simulink subsystem "BranchDecisionLogic"  (R2024b)
settings: Solver=VariableStepAuto  StartTime=0.0  StopTime=10.0  RelTol=1e-3
libraries: hdlsllib x1
settings Model: Creator=stefano  LastModifiedBy=stefano

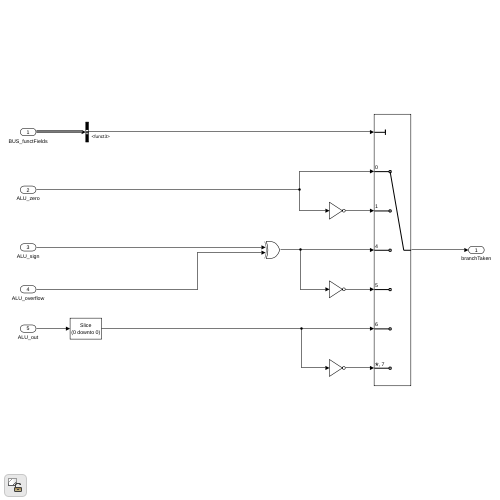
[thumbnail: Simulink's stored preview of the top-level diagram]
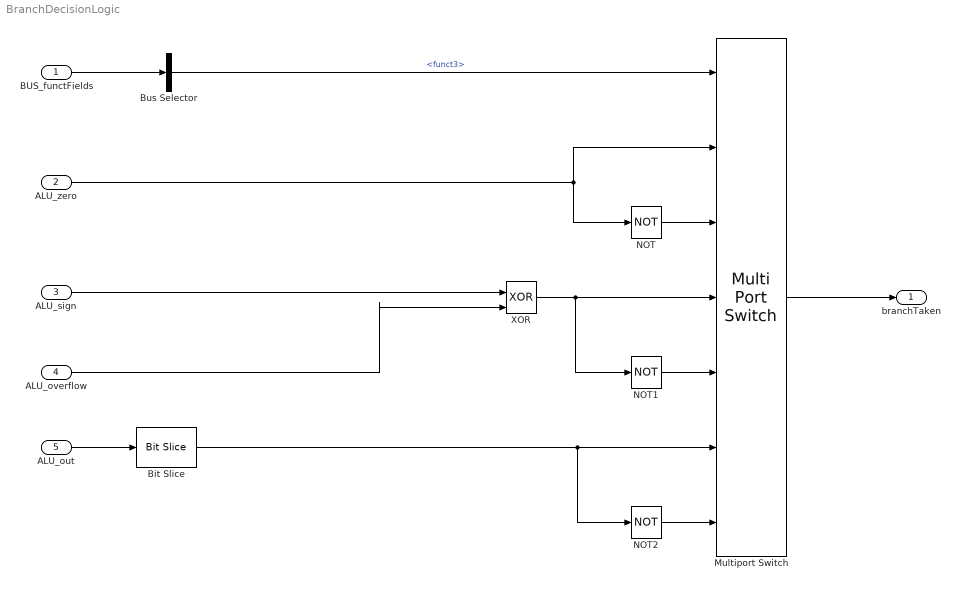
== system BranchDecisionLogic ==
  BUS_functFields : Inport
  ALU_zero : Inport  Port=2
  ALU_sign : Inport  Port=3
  ALU_overflow : Inport  Port=4
  ALU_out : Inport  Port=5
  Bit Slice : hdlsllib/Logic and Bit Operations/Bit Slice  lidx=0  ridx=0
  Bus Selector : BusSelector  OutputSignals=funct3
  Multiport Switch : MultiPortSwitch  DataPortOrder=Specify indices  DataPortIndices={0, 1, 4, 5, 6, 7}  DiagnosticForDefault=None  SaturateOnIntegerOverflow=off  InputSameDT=off
  NOT : Logic  Operator=NOT  IconShape=distinctive  AllPortsSameDT=off  OutDataTypeStr=boolean
  NOT1 : Logic  Operator=NOT  IconShape=distinctive  AllPortsSameDT=off  OutDataTypeStr=boolean
  NOT2 : Logic  Operator=NOT  IconShape=distinctive  AllPortsSameDT=off  OutDataTypeStr=boolean
  XOR : Logic  Operator=XOR  IconShape=distinctive  AllPortsSameDT=off  OutDataTypeStr=boolean
  branchTaken : Outport
  wires:
  BUS_functFields/1 -> Bus Selector/1
  Bus Selector/1 -> Multiport Switch/1  "<funct3>"
  Multiport Switch/1 -> branchTaken/1
  ALU_sign/1 -> XOR/1
  ALU_overflow/1 -> XOR/2
  ALU_zero/1 -> NOT/1, Multiport Switch/2
  NOT/1 -> Multiport Switch/3
  XOR/1 -> NOT1/1, Multiport Switch/4
  NOT1/1 -> Multiport Switch/5
  ALU_out/1 -> Bit Slice/1
  Bit Slice/1 -> Multiport Switch/6, NOT2/1
  NOT2/1 -> Multiport Switch/7
